simulink subsystem "heaviside"  (R2025b)
settings: Solver=VariableStepAuto  StartTime=0.0  StopTime=10.0  RelTol=1e-3
settings Model: Creator=sanborkl  LastModifiedBy=sanborkl

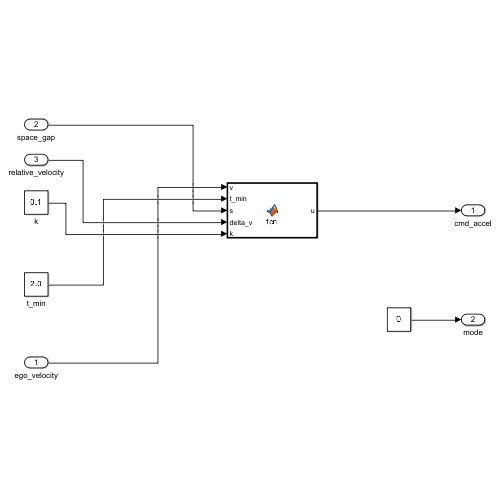
[thumbnail: Simulink's stored preview of the top-level diagram]
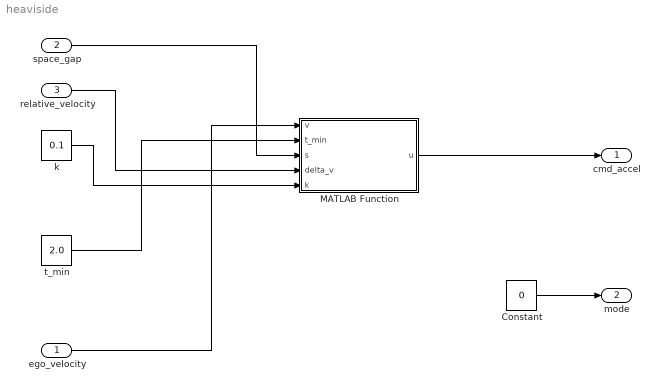
== system heaviside ==
  ego_velocity : Inport
  space_gap : Inport  Port=2
  relative_velocity : Inport  Port=3
  Constant : Constant  Value=0
  MATLAB Function : MATLAB Function  TreatAsAtomicUnit=on
  k : Constant  Value=0.1
  t_min : Constant  Value=2.0
  cmd_accel : Outport
  mode : Outport  Port=2
  wires:
  relative_velocity/1 -> MATLAB Function/4(delta_v)
  t_min/1 -> MATLAB Function/2(t_min)
  space_gap/1 -> MATLAB Function/3(s)
  ego_velocity/1 -> MATLAB Function/1(v)
  k/1 -> MATLAB Function/5(k)
  Constant/1 -> mode/1
  MATLAB Function/1(u) -> cmd_accel/1

== matlab function heaviside/MATLAB Function ==
  data: v input; u output; t_min input; s input; delta_v input; k input
function u = fcn(v, t_min, s, delta_v, k)

e_term = exp(2 * (v - 8.9));
fraction = 1 / (t_min + (20 * e_term)/((1 + e_term) ^ 2));

u = fraction * (delta_v + k * (s - ((t_min * v) + ((10 * e_term)/(1 + e_term)) + 5) ) );
